simulink model "Rate_AdapatingV2"  (R2023b)
settings: Solver=FixedStepAuto  StartTime=0.0  StopTime=15  FixedStep=1e-3  RelTol=1e-3  EnableMultiTasking=on
libraries: frdmk64flib x1, dspstat3 x1
settings Model: SimulationMode=external  ExtModeTrigDuration=5  Creator=Jeff  LastModifiedBy=conno
settings SolverCC: AlgebraicLoopSolver=TrustRegion
settings OptimizationCC: EnhancedBackFolding=on  PassReuseOutputArgsAs=Individual arguments  ZeroExternalMemoryAtStartup=off  ZeroInternalMemoryAtStartup=off  MaxStackSize=64  OptimizeBlockOrder=speed  DifferentSizesBufferReuse=on  OptimizationCustomize=off  EfficientTunableParamExpr=on
settings DebuggingCC: ParameterTunabilityLossMsg=error  UnconnectedInputMsg=warning  UnconnectedOutputMsg=warning  UnconnectedLineMsg=warning
settings HardwareCC: ProdBitPerPointer=32  ProdBitPerSizeT=32  ProdBitPerPtrDiffT=32  ProdLargestAtomicInteger=Long  ProdLargestAtomicFloat=Double  ProdWordSize=32  ProdHWDeviceType=ARM Compatible->ARM Cortex
settings ModelReferenceCC: EnableRefExpFcnMdlSchedulingChecks=on
settings RTWCC: Description=Embedded Coder  SystemTargetFile=ert.tlc  HardwareBoard=NXP FRDM-K64F  TLCOptions="-aInlineSetEventsForThisBaseRateFcn=TLC_FALSE -aSuppressMultiTaskScheduler=TLC_FALSE  -aRateBasedStepFcn=0"  TemplateMakefile=ert_default_tmf  Toolchain=GNU Tools for ARM Embedded Processors
settings CodeAppCC: ForceParamTrailComments=on  IgnoreCustomStorageClasses=off  OperatorAnnotations=on  SimulinkDataObjDesc=on  SFDataObjDesc=on  InsertBlockDesc=on
settings ERTTargetCC: SupportVariableSizeSignals=on

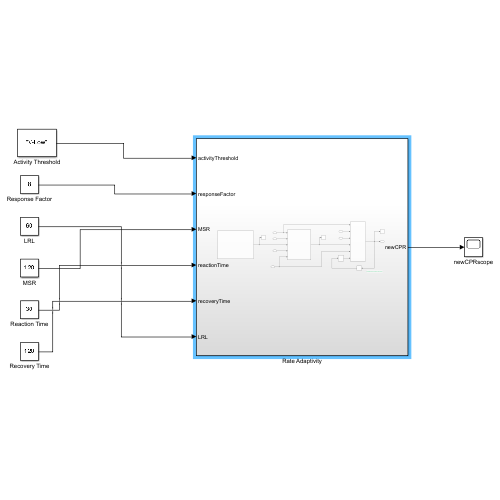
[thumbnail: Simulink's stored preview of the top-level diagram]
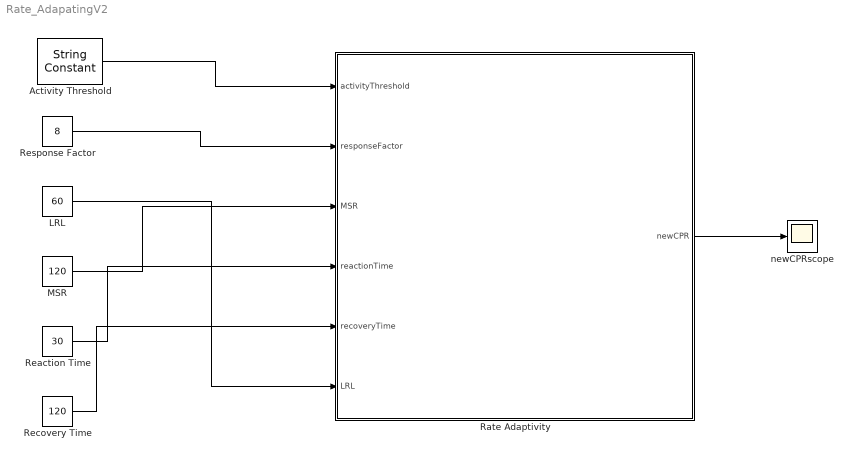
== system Rate_AdapatingV2 ==
  Activity Threshold : StringConstant  String="\"V-Low\""
  LRL : Constant  Value=60  OutDataTypeStr=double
  MSR : Constant  Value=120  OutDataTypeStr=double
  Rate Adaptivity : Subsystem
  Reaction Time : Constant  Value=30  OutDataTypeStr=double
  Recovery Time : Constant  Value=120  OutDataTypeStr=double
  Response Factor : Constant  Value=8  OutDataTypeStr=double
  newCPRscope : Scope
  wires:
  Activity Threshold/1 -> Rate Adaptivity/1(activityThreshold)
  Response Factor/1 -> Rate Adaptivity/2(responseFactor)
  LRL/1 -> Rate Adaptivity/6(LRL)
  MSR/1 -> Rate Adaptivity/3(MSR)
  Reaction Time/1 -> Rate Adaptivity/4(reactionTime)
  Recovery Time/1 -> Rate Adaptivity/5(recoveryTime)
  Rate Adaptivity/1(newCPR) -> newCPRscope/1

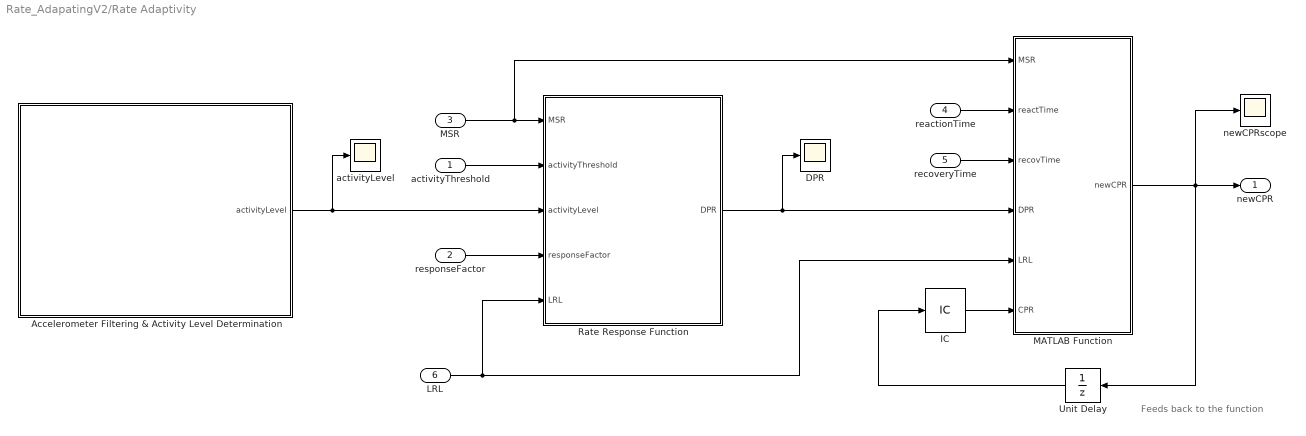
== system Rate_AdapatingV2/Rate Adaptivity ==
  note: Feeds back to the function
  activityThreshold : Inport
  responseFactor : Inport  Port=2
  MSR : Inport  Port=3
  reactionTime : Inport  Port=4
  recoveryTime : Inport  Port=5
  LRL : Inport  Port=6
  Accelerometer Filtering & Activity Level Determination : Subsystem
  DPR : Scope
  IC : InitialCondition  Value=60.0
  MATLAB Function : MATLAB Function  TreatAsAtomicUnit=on
  Rate Response Function : MATLAB Function  TreatAsAtomicUnit=on
  Unit Delay : UnitDelay  SampleTime=-1  HasFrameUpgradeWarning=on
  activityLevel : Scope
  newCPRscope : Scope
  newCPR : Outport
  wires:
  LRL/1 -> MATLAB Function/5(LRL), Rate Response Function/5(LRL)
  activityThreshold/1 -> Rate Response Function/2(activityThreshold)
  MSR/1 -> MATLAB Function/1(MSR), Rate Response Function/1(MSR)
  responseFactor/1 -> Rate Response Function/4(responseFactor)
  recoveryTime/1 -> MATLAB Function/3(recovTime)
  MATLAB Function/1(newCPR) -> Unit Delay/1, newCPR/1, newCPRscope/1
  reactionTime/1 -> MATLAB Function/2(reactTime)
  Rate Response Function/1(DPR) -> MATLAB Function/4(DPR), DPR/1
  Unit Delay/1 -> IC/1
  IC/1 -> MATLAB Function/6(CPR)
  Accelerometer Filtering & Activity Level Determination/1(activityLevel) -> Rate Response Function/3(activityLevel), activityLevel/1

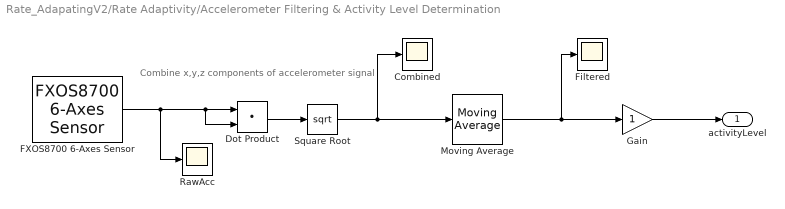
== system Rate_AdapatingV2/Rate Adaptivity/Accelerometer Filtering & Activity Level Determination ==
  note: Combine x,y,z components of accelerometer signal
  Combined : Scope
  Dot Product : DotProduct  OutDataTypeStr=Inherit: Inherit via internal rule
  FXOS8700 6-Axes Sensor : frdmk64flib/FXOS8700 6-Axes Sensor  Activesensor=Accelerometer only  ODR=800Hz  HybridODR=400Hz  Accelfullrange=-4g to +4g  SampleTime=-1
  Filtered : Scope
  Gain : Gain
  Moving Average : dspstat3/Moving Average  Method=Sliding window  ForgettingFactorPort=off  SpecifyWindowLength=on  WindowLength=4  OverlapLength=3  AllowArbitraryInputLength=off  ForgettingFactor=0.9  SimulateUsing=Code generation
  RawAcc : Scope
  Square Root : Sqrt
  activityLevel : Outport
  wires:
  Moving Average/1 -> Filtered/1, Gain/1
  Square Root/1 -> Moving Average/1, Combined/1
  Dot Product/1 -> Square Root/1
  FXOS8700 6-Axes Sensor/1 -> Dot Product/1, Dot Product/2, RawAcc/1
  Gain/1 -> activityLevel/1

== matlab function Rate_AdapatingV2/Rate Adaptivity/MATLAB Function ==
  data: MSR input; newCPR output; reactTime input; recovTime input; DPR input; LRL input; CPR input
function newCPR = timing(MSR, reactTime, recovTime, DPR, LRL, CPR)
if CPR < DPR % Increase Rate

    % Current Time based on Current Pace
    currTime = -log(1 - (LRL - CPR)/(LRL - MSR))*(reactTime/11 - 2/11);
    % Increase current time by 1ms
    currTime = currTime + 0.001;
    % New Pace Rate after 1ms increase
    newCPR = (1-exp(-11*currTime/(reactTime-2)))*(MSR-LRL) + LRL;

elseif CPR > DPR % Decrease Rate

    %Current Time based on Current Pace
    currTime = -log((LRL - CPR)/(LRL - MSR))*(recovTime/11 - 3/11);
    % Increase time by 1ms
    currTime = currTime + 0.001;
    %New Pace Rate after 1ms increase
    newCPR = (exp(-11*currTime/(recovTime-3)))*(MSR-LRL) + LRL;
      
else 
    newCPR = CPR; 

end
end

== matlab function Rate_AdapatingV2/Rate Adaptivity/Rate Response Function ==
  data: MSR input; activityThreshold input; DPR output; activityLevel input; responseFactor input; LRL input
function DPR  = fcn(MSR, activityThreshold, activityLevel, responseFactor, LRL)

% total range of change of acceleration 
ATMax = sqrt(4^2+4^2+4^2)-1; 

% since the accelerameter record the gravity (1g), 1g is removed to ensure when the pacemaker is static, there is no extra pacing 
activityThresholdLevels = {'V-Low', 'Low', 'Med-Low', 'Med', 'Med-High', 'High', 'V-High'}; %possible activity level string inputs

activityThresholdRange = [0.05*ATMax+1, 0.15*ATMax+1, 0.30*ATMax+1, 0.45*ATMax+1, 0.60*ATMax+1, 0.75*ATMax+1, 0.90*ATMax+1]; 
%take percentage of a maximum activity level, plus on to ensure the threshold is higher than defaul 1g (default acceleration reading

activityThresholdNum = activityThresholdRange(find(strcmp(activityThresholdLevels, char(activityThreshold)))); 
%map the string level of activity levels to a number value


if(activityLevel <= activityThresholdNum(1)) %doesn't meet the activity level threshold
    DPR = LRL;

elseif(activityLevel > activityThresholdNum(1) && activityLevel < sqrt(48))  % when the activity level is between threshold and max activity
    DPR = (1-exp((-(1/(sqrt(48)-activityLevel)*responseFactor*(activityLevel-activityThresholdNum(1))))))*(MSR-LRL)+LRL;

else
    DPR = MSR; %set to max sensor rate if activity level is greater than max activity

end
end
